simulink model "DFIG_FILTER"  (R2023a)
settings: Solver=ode23t  StartTime=0.0  StopTime=25  MaxStep=1e-6  RelTol=1e-3
model workspace (MAT data in the model file):
  Ts_phasor = 10
undefined symbols (not defined in the file): Base_Power, D1, Delta, F, find_system, Fnom, gcbh, H, ILd_init, ILq_init, Imax_grid_conv, Init, j, Ki_dc_reg, Ki_grid_side_cur_reg, Ki_power_reg, Ki_Q, Ki_rotor_side_cur_reg, Ki_volt_reg, Kp_dc_reg, Kp_grid_side_cur_reg, Kp_power_reg, Kp_Q, Kp_rotor_side_cur_reg, Kp_volt_reg, L_RL, Llr, Lls, p, Pnom, power_A, power_B, power_D, R_RL, Rr, Rs, speed_A, speed_B, speed_C, speed_D, sps_rtmsupport, Vcontrol, Vnom, Wind_On
libraries: spsPower3phPhasorLib x9, spsOnDelayLib x9, spsThreePhaseVIMeasurementLib x8, simulink_extras x5, spsRMSLib x4, spsControlledCurrentSourceLib x4, spsGroundLib x3, spsSeriesRLCBranchLib x2, spsThreePhaseSeriesRLCBranchLib x2, spspowerguiLib x2, spsThreePhasePISectionLineLib x2, spsThreePhaseTransformerTwoWindingsLib x2
(part 3 of 6)

== system DFIG_FILTER/MODEL (PHASER)/Wind turbine Data acquisition4/Mean Value2 ==
  note: Mean value
  In : Inport
  Init : Inport  Port=2
  Gain : Gain  Gain=1/Period  SaturateOnIntegerOverflow=on  OutDataTypeStr=Inherit: Same as input  ParamDataTypeStr=Inherit: Same as input
  Step : Step  Time=Period+eps  SampleTime=0
  Sum : Sum  Inputs=+-  InputSameDT=on  SaturateOnIntegerOverflow=on  OutDataTypeStr=Inherit: Same as first input
  Switch : Switch  Threshold=0.5  InputSameDT=off
  Transport Delay : TransportDelay  DelayTime=Period
  integrator : Integrator
  Mean : Outport  VectorParamsAs1DForOutWhenUnconnected=off
  wires:
  Init/1 -> Switch/3
  Step/1 -> Switch/2
  Switch/1 -> Mean/1
  Gain/1 -> Switch/1
  Sum/1 -> Gain/1
  In/1 -> integrator/1
  integrator/1 -> Sum/1, Transport Delay/1
  Transport Delay/1 -> Sum/2

== system DFIG_FILTER/MODEL (PHASER)/Wind turbine Data acquisition4/magnitude positive seq.  ==
  In1 : Inport
  Complex to Real-Imag : ComplexToRealImag
  Fourier1 : Subsystem  mask(Fourier analyser){f1=60, n=0}
      mask prompts: f1 "Fundamental frequency f1 (Hz):"; n "Harmonic n (0=DC; 1=fundamental; 2=2nd harm;  ...) :"
      mask help: The Fourier block performs a Fourier analysis of the input signal over a running window of one cycle of the fundamental frequency. First and second outputs return respectively the magnitude and phase (degrees) of the harmonic component specified.
      mask init:
      | k=2-(n==0);
      mask Help: helpview(psbhelp)
  Fourier2 : Subsystem  mask(Fourier analyser){f1=60, n=0}
      mask prompts: f1 "Fundamental frequency f1 (Hz):"; n "Harmonic n (0=DC; 1=fundamental; 2=2nd harm;  ...) :"
      mask help: The Fourier block performs a Fourier analysis of the input signal over a running window of one cycle of the fundamental frequency. First and second outputs return respectively the magnitude and phase (degrees) of the harmonic component specified.
      mask init:
      | k=2-(n==0);
      mask Help: helpview(psbhelp)
  Math Function : Math  Operator=hypot  SignedPower=on
  Terminator : Terminator
  Terminator1 : Terminator
  Out1 : Outport  VectorParamsAs1DForOutWhenUnconnected=off
  wires:
  In1/1 -> Complex to Real-Imag/1
  Math Function/1 -> Out1/1
  Fourier2/1(magnitude) -> Math Function/2
  Fourier1/1(magnitude) -> Math Function/1
  Fourier2/2(angle) -> Terminator1/1
  Fourier1/2(angle) -> Terminator/1
  Complex to Real-Imag/2 -> Fourier2/1(signal)
  Complex to Real-Imag/1 -> Fourier1/1(signal)

== system DFIG_FILTER/MODEL (PHASER)/Wind turbine Data acquisition4/magnitude positivie seq ==
  In1 : Inport
  Complex to Real-Imag : ComplexToRealImag
  Fourier1 : Subsystem  mask(Fourier analyser){f1=60, n=0}
      mask prompts: f1 "Fundamental frequency f1 (Hz):"; n "Harmonic n (0=DC; 1=fundamental; 2=2nd harm;  ...) :"
      mask help: The Fourier block performs a Fourier analysis of the input signal over a running window of one cycle of the fundamental frequency. First and second outputs return respectively the magnitude and phase (degrees) of the harmonic component specified.
      mask init:
      | k=2-(n==0);
      mask Help: helpview(psbhelp)
  Fourier2 : Subsystem  mask(Fourier analyser){f1=60, n=0}
      mask prompts: f1 "Fundamental frequency f1 (Hz):"; n "Harmonic n (0=DC; 1=fundamental; 2=2nd harm;  ...) :"
      mask help: The Fourier block performs a Fourier analysis of the input signal over a running window of one cycle of the fundamental frequency. First and second outputs return respectively the magnitude and phase (degrees) of the harmonic component specified.
      mask init:
      | k=2-(n==0);
      mask Help: helpview(psbhelp)
  Math Function : Math  Operator=hypot  SignedPower=on
  Terminator : Terminator
  Terminator1 : Terminator
  Out1 : Outport  VectorParamsAs1DForOutWhenUnconnected=off
  wires:
  Complex to Real-Imag/1 -> Fourier1/1(signal)
  Complex to Real-Imag/2 -> Fourier2/1(signal)
  Fourier1/2(angle) -> Terminator/1
  Fourier2/2(angle) -> Terminator1/1
  Fourier1/1(magnitude) -> Math Function/1
  Fourier2/1(magnitude) -> Math Function/2
  Math Function/1 -> Out1/1
  In1/1 -> Complex to Real-Imag/1

== system DFIG_FILTER/MODEL (PHASER)/Wind turbine Data acquisition5/Mean Value1 ==
  note: Mean value
  In : Inport
  Init : Inport  Port=2
  Gain : Gain  Gain=1/Period  SaturateOnIntegerOverflow=on  OutDataTypeStr=Inherit: Same as input  ParamDataTypeStr=Inherit: Same as input
  Step : Step  Time=Period+eps  SampleTime=0
  Sum : Sum  Inputs=+-  InputSameDT=on  SaturateOnIntegerOverflow=on  OutDataTypeStr=Inherit: Same as first input
  Switch : Switch  Threshold=0.5  InputSameDT=off
  Transport Delay : TransportDelay  DelayTime=Period
  integrator : Integrator
  Mean : Outport  VectorParamsAs1DForOutWhenUnconnected=off
  wires:
  Transport Delay/1 -> Sum/2
  integrator/1 -> Transport Delay/1, Sum/1
  In/1 -> integrator/1
  Sum/1 -> Gain/1
  Gain/1 -> Switch/1
  Switch/1 -> Mean/1
  Step/1 -> Switch/2
  Init/1 -> Switch/3

== system DFIG_FILTER/MODEL (PHASER)/Wind turbine Data acquisition5/Mean Value2 ==
  note: Mean value
  In : Inport
  Init : Inport  Port=2
  Gain : Gain  Gain=1/Period  SaturateOnIntegerOverflow=on  OutDataTypeStr=Inherit: Same as input  ParamDataTypeStr=Inherit: Same as input
  Step : Step  Time=Period+eps  SampleTime=0
  Sum : Sum  Inputs=+-  InputSameDT=on  SaturateOnIntegerOverflow=on  OutDataTypeStr=Inherit: Same as first input
  Switch : Switch  Threshold=0.5  InputSameDT=off
  Transport Delay : TransportDelay  DelayTime=Period
  integrator : Integrator
  Mean : Outport  VectorParamsAs1DForOutWhenUnconnected=off
  wires:
  Init/1 -> Switch/3
  Step/1 -> Switch/2
  Switch/1 -> Mean/1
  Gain/1 -> Switch/1
  Sum/1 -> Gain/1
  In/1 -> integrator/1
  integrator/1 -> Sum/1, Transport Delay/1
  Transport Delay/1 -> Sum/2

== system DFIG_FILTER/MODEL (PHASER)/Wind turbine Data acquisition5/magnitude positive seq.  ==
  In1 : Inport
  Complex to Real-Imag : ComplexToRealImag
  Fourier1 : Subsystem  mask(Fourier analyser){f1=60, n=0}
      mask prompts: f1 "Fundamental frequency f1 (Hz):"; n "Harmonic n (0=DC; 1=fundamental; 2=2nd harm;  ...) :"
      mask help: The Fourier block performs a Fourier analysis of the input signal over a running window of one cycle of the fundamental frequency. First and second outputs return respectively the magnitude and phase (degrees) of the harmonic component specified.
      mask init:
      | k=2-(n==0);
      mask Help: helpview(psbhelp)
  Fourier2 : Subsystem  mask(Fourier analyser){f1=60, n=0}
      mask prompts: f1 "Fundamental frequency f1 (Hz):"; n "Harmonic n (0=DC; 1=fundamental; 2=2nd harm;  ...) :"
      mask help: The Fourier block performs a Fourier analysis of the input signal over a running window of one cycle of the fundamental frequency. First and second outputs return respectively the magnitude and phase (degrees) of the harmonic component specified.
      mask init:
      | k=2-(n==0);
      mask Help: helpview(psbhelp)
  Math Function : Math  Operator=hypot  SignedPower=on
  Terminator : Terminator
  Terminator1 : Terminator
  Out1 : Outport  VectorParamsAs1DForOutWhenUnconnected=off
  wires:
  In1/1 -> Complex to Real-Imag/1
  Math Function/1 -> Out1/1
  Fourier2/1(magnitude) -> Math Function/2
  Fourier1/1(magnitude) -> Math Function/1
  Fourier2/2(angle) -> Terminator1/1
  Fourier1/2(angle) -> Terminator/1
  Complex to Real-Imag/2 -> Fourier2/1(signal)
  Complex to Real-Imag/1 -> Fourier1/1(signal)

== system DFIG_FILTER/MODEL (PHASER)/Wind turbine Data acquisition5/magnitude positivie seq ==
  In1 : Inport
  Complex to Real-Imag : ComplexToRealImag
  Fourier1 : Subsystem  mask(Fourier analyser){f1=60, n=0}
      mask prompts: f1 "Fundamental frequency f1 (Hz):"; n "Harmonic n (0=DC; 1=fundamental; 2=2nd harm;  ...) :"
      mask help: The Fourier block performs a Fourier analysis of the input signal over a running window of one cycle of the fundamental frequency. First and second outputs return respectively the magnitude and phase (degrees) of the harmonic component specified.
      mask init:
      | k=2-(n==0);
      mask Help: helpview(psbhelp)
  Fourier2 : Subsystem  mask(Fourier analyser){f1=60, n=0}
      mask prompts: f1 "Fundamental frequency f1 (Hz):"; n "Harmonic n (0=DC; 1=fundamental; 2=2nd harm;  ...) :"
      mask help: The Fourier block performs a Fourier analysis of the input signal over a running window of one cycle of the fundamental frequency. First and second outputs return respectively the magnitude and phase (degrees) of the harmonic component specified.
      mask init:
      | k=2-(n==0);
      mask Help: helpview(psbhelp)
  Math Function : Math  Operator=hypot  SignedPower=on
  Terminator : Terminator
  Terminator1 : Terminator
  Out1 : Outport  VectorParamsAs1DForOutWhenUnconnected=off
  wires:
  Complex to Real-Imag/1 -> Fourier1/1(signal)
  Complex to Real-Imag/2 -> Fourier2/1(signal)
  Fourier1/2(angle) -> Terminator/1
  Fourier2/2(angle) -> Terminator1/1
  Fourier1/1(magnitude) -> Math Function/1
  Fourier2/1(magnitude) -> Math Function/2
  Math Function/1 -> Out1/1
  In1/1 -> Complex to Real-Imag/1

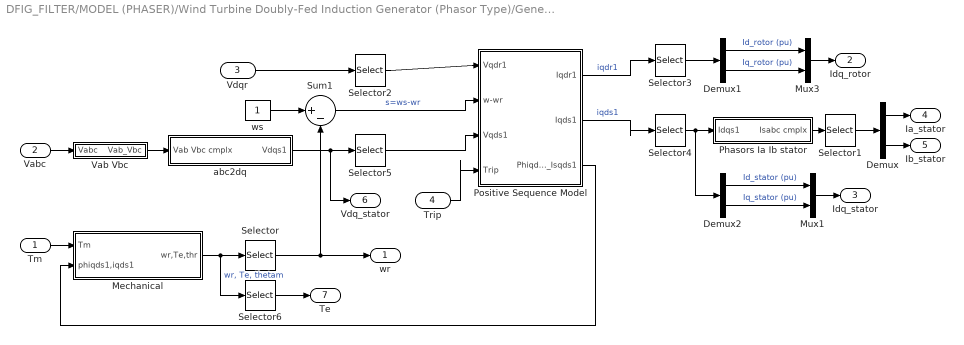
== system DFIG_FILTER/MODEL (PHASER)/Wind Turbine Doubly-Fed Induction Generator (Phasor Type)/Generator & Converters/Asynchronous machine Positive sequence phasor model Inputs and outputs are in per unit (pu) ==
  Tm : Inport
  Vabc : Inport  Port=2
  "Vdqr " : Inport  Port=3
  Trip : Inport  Port=4
  Demux : Demux  Outputs=2
      settings: DisplayOption=none
  Demux1 : Demux  Outputs=2
      settings: DisplayOption=none
  Demux2 : Demux  Outputs=2
      settings: DisplayOption=none
  Mechanical : Subsystem
  Mux1 : Mux  Inputs=2
  Mux3 : Mux  Inputs=2
  Phasors Ia Ib stator : Subsystem
  Positive Sequence Model : Subsystem
  Selector : Selector  InputPortWidth=3  IndexOptions=Index vector (dialog)  Indices=1  OutputSizes=1
  Selector1 : Selector  InputPortWidth=3  IndexOptions=Index vector (dialog)  Indices=[1 2]  OutputSizes=1
  Selector{2..5} (4 alike) : Selector  InputPortWidth=2  IndexOptions=Index vector (dialog)  Indices=[2 1]  OutputSizes=1
  Selector6 : Selector  InputPortWidth=3  IndexOptions=Index vector (dialog)  Indices=2  OutputSizes=1
  Sum1 : Sum  Inputs=|+-  InputSameDT=on  SaturateOnIntegerOverflow=on  OutDataTypeStr=Inherit: Same as first input
  Vab Vbc : Subsystem
  abc2dq : Subsystem
  ws : Constant
  wr : Outport  VectorParamsAs1DForOutWhenUnconnected=off
  Idq_rotor : Outport  Port=2  VectorParamsAs1DForOutWhenUnconnected=off
  Idq_stator : Outport  Port=3  VectorParamsAs1DForOutWhenUnconnected=off
  Ia_stator : Outport  Port=4  VectorParamsAs1DForOutWhenUnconnected=off
  Ib_stator : Outport  Port=5  VectorParamsAs1DForOutWhenUnconnected=off
  Vdq_stator : Outport  Port=6  VectorParamsAs1DForOutWhenUnconnected=off
  Te : Outport  Port=7  VectorParamsAs1DForOutWhenUnconnected=off
  wires:
  Selector4/1 -> Phasors Ia Ib stator/1(Idqs1), Demux2/1
  Selector5/1 -> Positive Sequence Model/3(Vqds1)
  Selector2/1 -> Positive Sequence Model/1(Vqdr1)
  Sum1/1 -> Positive Sequence Model/2(w-wr)  "s=ws-wr"
  Selector/1 -> wr/1, Sum1/2
  ws/1 -> Sum1/1
  Mechanical/1(wr,Te,thr) -> Selector/1, Selector6/1  "wr, Te, thetam"
  "Vdqr "/1 -> Selector2/1
  abc2dq/1(Vdqs1) -> Selector5/1, Vdq_stator/1
  Vab Vbc/1(Vab_Vbc) -> abc2dq/1(Vab Vbc cmplx)
  Vabc/1 -> Vab Vbc/1(Vabc)
  Phasors Ia Ib stator/1(Isabc cmplx) -> Selector1/1
  Tm/1 -> Mechanical/1(Tm)
  Demux/1 -> Ia_stator/1
  Demux/2 -> Ib_stator/1
  Selector1/1 -> Demux/1
  Selector6/1 -> Te/1
  Selector3/1 -> Demux1/1
  Demux1/1 -> Mux3/1  "Id_rotor (pu)"
  Demux1/2 -> Mux3/2  "Iq_rotor (pu)"
  Mux3/1 -> Idq_rotor/1
  Demux2/1 -> Mux1/1  "Id_stator (pu)"
  Demux2/2 -> Mux1/2  "Iq_stator (pu)"
  Mux1/1 -> Idq_stator/1
  Positive Sequence Model/1(Iqdr1) -> Selector3/1  "iqdr1"
  Positive Sequence Model/2(Iqds1) -> Selector4/1  "iqds1"
  Positive Sequence Model/3(Phiqds1_Isqds1) -> Mechanical/2(phiqds1,iqds1)
  Trip/1 -> Positive Sequence Model/4(Trip)

== system DFIG_FILTER/MODEL (PHASER)/Wind Turbine Doubly-Fed Induction Generator (Phasor Type)/Generator & Converters/Control ==
  Vabc_B1 : Inport
  Idq_grid_conv : Inport  Port=2
  Vdc : Inport  Port=3
  wr : Inport  Port=4
  Idq_stator : Inport  Port=5
  Idq_rotor : Inport  Port=6
  V_ref : Inport  Port=7  SampleTime=0
  Q_ref : Inport  Port=8  SampleTime=0
  Iq_grid_conv_ref : Inport  Port=9  SampleTime=0
  P_B1 : Inport  Port=10
  Q_B1 : Inport  Port=11
  Trip : Inport  Port=12
  0-inf : Saturate  UpperLimit=inf  LowerLimit=0
  0-pitch_max : Saturate  UpperLimit=pitch_max  LowerLimit=0
  Constant2 : Constant  Value=speed_D
  Converters voltages : Subsystem
  Logical Operator : Logic  Operator=NOT  AllPortsSameDT=off  OutDataTypeStr=float('double')  SampleTime=0
  Power(speed) : Lookup_n-D  NumberOfTableDimensions=1  BreakpointsForDimension1=speed_power(:,1)  Table=speed_power(:,2)  InternalRulePriority=Speed  RndMeth=Simplest
  "Rate Limiter " : RateLimiter  RisingSlewLimit=power_slew_rate  FallingSlewLimit=-power_slew_rate
  "Rate Limiter   " : RateLimiter  RisingSlewLimit=pitch_rate  FallingSlewLimit=-pitch_rate
  Sum : Sum  Inputs=|+-  SaturateOnIntegerOverflow=on
  abc2dq & Positive sequence Voltage phase angle : Subsystem
  pitch_gain : Gain  Gain=pitch_gain  SaturateOnIntegerOverflow=on  OutDataTypeStr=Inherit: Same as input  ParamDataTypeStr=Inherit: Same as input
  wind_dfig_grid : Subsystem
  wind_dfig_rotor : Subsystem
  Vdq_rotor_conv : Outport  VectorParamsAs1DForOutWhenUnconnected=off
  Vdq_B1 : Outport  Port=2  VectorParamsAs1DForOutWhenUnconnected=off
  Vdq_grid_conv : Outport  Port=3  VectorParamsAs1DForOutWhenUnconnected=off
  Pitch_angle : Outport  Port=4  VectorParamsAs1DForOutWhenUnconnected=off
  wires:
  Vdc/1 -> Converters voltages/2(Vdc), wind_dfig_grid/4(Vdc), wind_dfig_rotor/2(Vdc)
  abc2dq & Positive sequence Voltage phase angle/2(Theta) -> wind_dfig_grid/3(Theta), wind_dfig_rotor/3(Theta)
  abc2dq & Positive sequence Voltage phase angle/1(Vdq_B1) -> Vdq_B1/1, wind_dfig_grid/1(Vdq_B1)
  Converters voltages/2(Vdq_rotor_conv) -> Vdq_rotor_conv/1
  Converters voltages/1(Vdq_grid_conv) -> Vdq_grid_conv/1
  Idq_grid_conv/1 -> wind_dfig_grid/2(Idq_grid_conv), wind_dfig_rotor/11(Idq_grid_conv)
  Vabc_B1/1 -> abc2dq & Positive sequence Voltage phase angle/1(Vabc_B1)
  Iq_grid_conv_ref/1 -> wind_dfig_grid/5(Iq_ref)
  Idq_stator/1 -> wind_dfig_rotor/4(Idq_stator)
  Idq_rotor/1 -> wind_dfig_rotor/5(Idq_rotor)
  V_ref/1 -> wind_dfig_rotor/6(V_ref)
  Q_ref/1 -> wind_dfig_rotor/7(Q_ref)
  abc2dq & Positive sequence Voltage phase angle/3(V_B1) -> wind_dfig_rotor/8(V_B1)
  wr/1 -> Power(speed)/1, Sum/1, wind_dfig_rotor/1(wr)
  P_B1/1 -> wind_dfig_rotor/9(P_B1)
  Q_B1/1 -> wind_dfig_rotor/10(Q_B1)
  Trip/1 -> Logical Operator/1
  wind_dfig_grid/1(Vdq_ctrl_grid_conv) -> Converters voltages/1(Vdq_ctrl_grid_conv)
  0-inf/1 -> "Rate Limiter "/1
  Power(speed)/1 -> 0-inf/1
  "Rate Limiter "/1 -> wind_dfig_rotor/12(Power_opt)
  0-pitch_max/1 -> "Rate Limiter   "/1
  Constant2/1 -> Sum/2
  Sum/1 -> pitch_gain/1
  pitch_gain/1 -> 0-pitch_max/1
  "Rate Limiter   "/1 -> Pitch_angle/1
  wind_dfig_rotor/1(Vdq_ctrl_rotor_conv) -> Converters voltages/3(Vdq_ctrl_rotor_conv)
  Logical Operator/1 -> wind_dfig_grid/Enable, wind_dfig_rotor/Enable

== system DFIG_FILTER/MODEL (PHASER)/Wind Turbine Doubly-Fed Induction Generator (Phasor Type)/Generator & Converters/DC bus model ==
  note: Pdc = Pac_grid_conv - Pac_rotor_conv
  Pac_grid_conv : Inport
  Pac_rotor_conv : Inport  Port=2
  Integrator : Integrator  InitialCondition=Vdc_Init  LowerSaturationLimit=1e-6  ZeroCross=off
  Product2 : Product  Inputs=*/  InputSameDT=on  SaturateOnIntegerOverflow=on  OutDataTypeStr=Inherit: Same as first input
  Sum2 : Sum  Inputs=|+-  InputSameDT=on  SaturateOnIntegerOverflow=on  OutDataTypeStr=Inherit: Same as first input
  deg->rad1 : Gain  Gain=1/C  SaturateOnIntegerOverflow=on  OutDataTypeStr=Inherit: Same as input  ParamDataTypeStr=Inherit: Same as input
  pu->W : Gain  Gain=Pnom  SaturateOnIntegerOverflow=on  OutDataTypeStr=Inherit: Same as input  ParamDataTypeStr=Inherit: Same as input
  Vdc : Outport  VectorParamsAs1DForOutWhenUnconnected=off
  wires:
  pu->W/1 -> Product2/1
  Pac_grid_conv/1 -> Sum2/1
  deg->rad1/1 -> Integrator/1
  Integrator/1 -> Vdc/1, Product2/2  "Vdc"
  Product2/1 -> deg->rad1/1  "Idc"
  Pac_rotor_conv/1 -> Sum2/2
  Sum2/1 -> pu->W/1

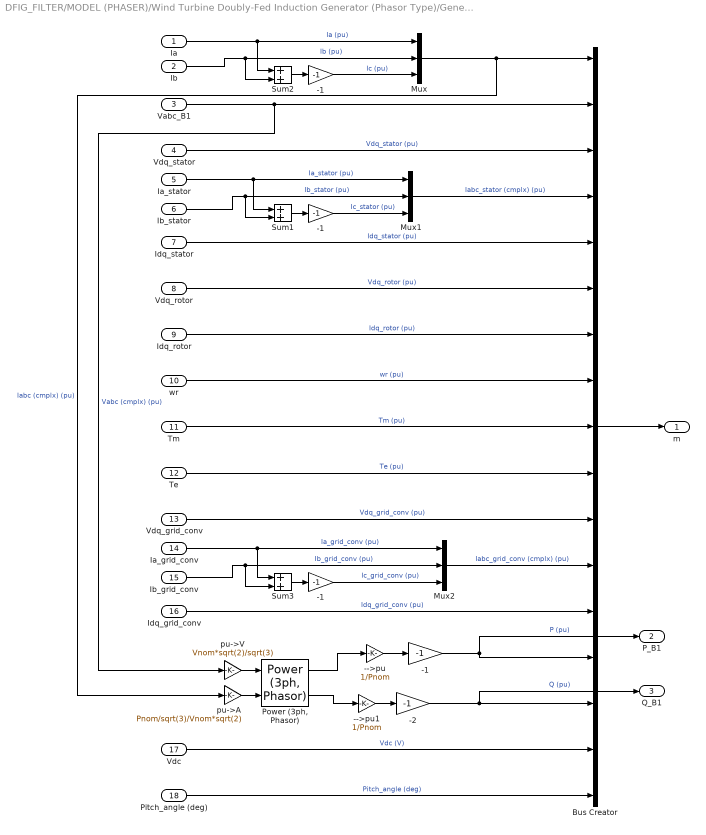
== system DFIG_FILTER/MODEL (PHASER)/Wind Turbine Doubly-Fed Induction Generator (Phasor Type)/Generator & Converters/Data acquisition ==
  Ia : Inport
  Ib : Inport  Port=2
  Vabc_B1 : Inport  Port=3
  Vdq_stator : Inport  Port=4
  Ia_stator : Inport  Port=5
  Ib_stator : Inport  Port=6
  Idq_stator : Inport  Port=7
  Vdq_rotor : Inport  Port=8
  Idq_rotor : Inport  Port=9
  wr : Inport  Port=10
  Tm : Inport  Port=11
  Te : Inport  Port=12
  Vdq_grid_conv : Inport  Port=13
  Ia_grid_conv : Inport  Port=14
  Ib_grid_conv : Inport  Port=15
  Idq_grid_conv : Inport  Port=16
  Vdc : Inport  Port=17
  Pitch_angle (deg) : Inport  Port=18
  " -1" : Gain  Gain=-1  SaturateOnIntegerOverflow=on  OutDataTypeStr=Inherit: Same as input  ParamDataTypeStr=Inherit: Same as input
  -->pu : Gain  Gain=1/Pnom  SaturateOnIntegerOverflow=on  OutDataTypeStr=Inherit: Same as input  ParamDataTypeStr=Inherit: Same as input
  -->pu1 : Gain  Gain=1/Pnom  SaturateOnIntegerOverflow=on  OutDataTypeStr=Inherit: Same as input  ParamDataTypeStr=Inherit: Same as input
  -1 : Gain  Gain=-1  SaturateOnIntegerOverflow=on  OutDataTypeStr=Inherit: Same as input  ParamDataTypeStr=Inherit: Same as input
  "-1 " : Gain  Gain=-1  SaturateOnIntegerOverflow=on  OutDataTypeStr=Inherit: Same as input  ParamDataTypeStr=Inherit: Same as input
  "-1  " : Gain  Gain=-1  SaturateOnIntegerOverflow=on  OutDataTypeStr=Inherit: Same as input  ParamDataTypeStr=Inherit: Same as input
  -2 : Gain  Gain=-1  SaturateOnIntegerOverflow=on  OutDataTypeStr=Inherit: Same as input  ParamDataTypeStr=Inherit: Same as input
  Bus Creator : BusCreator  Inputs=17
  Mux : Mux  Inputs=3
  Mux1 : Mux  Inputs=3
  Mux2 : Mux  Inputs=3
  "Power (3ph, Phasor)" : spsPower3phPhasorLib/Power (3ph, Phasor)
      settings: LibrarySourceBlock=|
      | sps_lib/Sensors and Measurements/Power
      | (3ph, Phasor)
  Sum1 : Sum  SaturateOnIntegerOverflow=on
  Sum2 : Sum  SaturateOnIntegerOverflow=on
  Sum3 : Sum  SaturateOnIntegerOverflow=on
  pu->A : Gain  Gain=Pnom/sqrt(3)/Vnom*sqrt(2)  SaturateOnIntegerOverflow=on  OutDataTypeStr=Inherit: Same as input  ParamDataTypeStr=Inherit: Same as input
  pu->V : Gain  Gain=Vnom*sqrt(2)/sqrt(3)  SaturateOnIntegerOverflow=on  OutDataTypeStr=Inherit: Same as input  ParamDataTypeStr=Inherit: Same as input
  m : Outport  VectorParamsAs1DForOutWhenUnconnected=off
  P_B1 : Outport  Port=2  VectorParamsAs1DForOutWhenUnconnected=off
  Q_B1 : Outport  Port=3  VectorParamsAs1DForOutWhenUnconnected=off
  wires:
  pu->A/1 -> "Power (3ph, Phasor)"/2
  -->pu/1 -> -1/1
  Sum2/1 -> "-1 "/1
  "-1 "/1 -> Mux/3  "Ic (pu)"
  Ib/1 -> Sum2/2, Mux/2  "Ib (pu)"
  Ia/1 -> Sum2/1, Mux/1  "Ia (pu)"
  Sum1/1 -> "-1  "/1
  "-1  "/1 -> Mux1/3  "Ic_stator (pu)"
  Ib_stator/1 -> Mux1/2, Sum1/2  "Ib_stator (pu)"
  Ia_stator/1 -> Mux1/1, Sum1/1  "Ia_stator (pu)"
  pu->V/1 -> "Power (3ph, Phasor)"/1
  Sum3/1 -> " -1"/1
  " -1"/1 -> Mux2/3  "Ic_grid_conv (pu)"
  Ib_grid_conv/1 -> Sum3/2, Mux2/2  "Ib_grid_conv (pu)"
  Ia_grid_conv/1 -> Sum3/1, Mux2/1  "Ia_grid_conv (pu)"
  Mux1/1 -> Bus Creator/4  "Iabc_stator (cmplx) (pu)"
  Mux/1 -> pu->A/1, Bus Creator/1  "Iabc (cmplx) (pu)"
  Vabc_B1/1 -> pu->V/1, Bus Creator/2  "Vabc (cmplx) (pu)"
  Vdq_stator/1 -> Bus Creator/3  "Vdq_stator (pu)"
  Idq_stator/1 -> Bus Creator/5  "Idq_stator (pu)"
  Vdq_rotor/1 -> Bus Creator/6  "Vdq_rotor (pu)"
  Idq_rotor/1 -> Bus Creator/7  "Idq_rotor (pu)"
  wr/1 -> Bus Creator/8  "wr (pu)"
  Tm/1 -> Bus Creator/9  "Tm (pu)"
  Te/1 -> Bus Creator/10  "Te (pu)"
  Vdq_grid_conv/1 -> Bus Creator/11  "Vdq_grid_conv (pu)"
  Mux2/1 -> Bus Creator/12  "Iabc_grid_conv (cmplx) (pu)"
  Idq_grid_conv/1 -> Bus Creator/13  "Idq_grid_conv (pu)"
  Vdc/1 -> Bus Creator/16  "Vdc (V)"
  -2/1 -> Q_B1/1, Bus Creator/15  "Q (pu)"
  -1/1 -> Bus Creator/14, P_B1/1  "P (pu)"
  Pitch_angle (deg)/1 -> Bus Creator/17  "Pitch_angle (deg)"
  Bus Creator/1 -> m/1
  -->pu1/1 -> -2/1
  "Power (3ph, Phasor)"/1 -> -->pu/1
  "Power (3ph, Phasor)"/2 -> -->pu1/1

== system DFIG_FILTER/MODEL (PHASER)/Wind Turbine Doubly-Fed Induction Generator (Phasor Type)/Generator & Converters/Grid-side converter currents & Converters power ==
  Vdq_rotor_conv : Inport
  Vdq_B1 : Inport  Port=2
  Vdq_grid_conv : Inport  Port=3
  Idq_rotor_conv : Inport  Port=4
  Trip : Inport  Port=5
  Demux : Demux  Outputs=2
      settings: DisplayOption=none
  Demux1 : Demux  Outputs=2
      settings: DisplayOption=none
  Mux2 : Mux  Inputs=2
  Product1 : Product  Inputs=**  InputSameDT=on  SaturateOnIntegerOverflow=on  OutDataTypeStr=Inherit: Same as first input
  Product3 : Product  Inputs=**  InputSameDT=on  SaturateOnIntegerOverflow=on  OutDataTypeStr=Inherit: Same as first input
  Sum1 : Sum  Inputs=1  InputSameDT=on  SaturateOnIntegerOverflow=on  OutDataTypeStr=Inherit: Same as first input
  Sum3 : Sum  Inputs=1  InputSameDT=on  SaturateOnIntegerOverflow=on  OutDataTypeStr=Inherit: Same as first input
  d-q axis model of a 3-phase series R-L branch : Subsystem  mask(d-q axis model of a 3-phase series R-L branch){R=R_RL, L=L_RL, Fnom=Fnom, Idq0=[ILd_init ILq_init]}
      mask prompts: R "R (pu)"; L "L (pu)"; Fnom "Nominal frequency (Hz)"; Idq0 "Initial currents [Id Iq] (pu)"
      mask help:
      | This block implements a d-q axis model of a 3-phase R-L branch.
      | Inputs:
      | d-q axis voltages (V1 and V2) at each terminal of the R-L branch in pu.
      | Outputs:
      | d-q axis currents flowing (from V1 to V2) in the R-L branch in pu.
      mask init:
      | w=2*pi*Fnom;
  dq2ab : Subsystem
  Ia_grid_conv : Outport  VectorParamsAs1DForOutWhenUnconnected=off
  Ib_grid_conv : Outport  Port=2  VectorParamsAs1DForOutWhenUnconnected=off
  Idq_grid_conv : Outport  Port=3  VectorParamsAs1DForOutWhenUnconnected=off
  Pac_grid_conv : Outport  Port=4  VectorParamsAs1DForOutWhenUnconnected=off
  Pac_rotor_conv : Outport  Port=5  VectorParamsAs1DForOutWhenUnconnected=off
  wires:
  Demux/2 -> Ib_grid_conv/1
  Demux/1 -> Ia_grid_conv/1
  dq2ab/1(Ia_Ib complx) -> Demux/1
  d-q axis model of a 3-phase series R-L branch/1(Idq) -> dq2ab/1(Idq_seq1), Demux1/1, Product3/1
  Idq_rotor_conv/1 -> Product1/2
  Vdq_rotor_conv/1 -> Product1/1
  Sum1/1 -> Pac_rotor_conv/1
  Product1/1 -> Sum1/1
  Sum3/1 -> Pac_grid_conv/1
  Product3/1 -> Sum3/1
  Vdq_grid_conv/1 -> d-q axis model of a 3-phase series R-L branch/2(Vdq2), Product3/2
  Vdq_B1/1 -> d-q axis model of a 3-phase series R-L branch/1(Vdq1)
  Demux1/1 -> Mux2/1  "Id_grid_conv (pu)"
  Demux1/2 -> Mux2/2  "Iq_grid_conv (pu)"
  Mux2/1 -> Idq_grid_conv/1
  Trip/1 -> d-q axis model of a 3-phase series R-L branch/3(Trip)

== system DFIG_FILTER/MODEL (PHASER)/Wind Turbine Protection/Protection System/AC Current Protection ==
  abc : Inport  PortDimensions=3
  Complex to Magnitude-Angle1 : ComplexToMagnitudeAngle  Output=Magnitude
  Current Measurement : Subsystem
  MinMax : MinMax  Function=max  InputSameDT=on  SaturateOnIntegerOverflow=on  ZeroCross=off
  Mux : Mux  Inputs=3
  On Delay : spsOnDelayLib/On Delay  DelayType=On delay  delay=Delay_I1  ic=0  Ts=0
  On Delay1 : spsOnDelayLib/On Delay  DelayType=On delay  delay=Delay_I2_I1  ic=0  Ts=0
  Relational Operator10 : RelationalOperator  Operator=>  InputSameDT=off
  Relational Operator6 : RelationalOperator  Operator=>  InputSameDT=off
  Relational Operator8 : RelationalOperator  Operator=>  InputSameDT=off
  Selector : Selector  InputPortWidth=3  IndexOptions=Index vector (dialog)  Indices=1  OutputSizes=1
  Selector1 : Selector  InputPortWidth=3  IndexOptions=Index vector (dialog)  Indices=2  OutputSizes=1
  Selector2 : Selector  InputPortWidth=3  IndexOptions=Index vector (dialog)  Indices=3  OutputSizes=1
  V0/V1 max3 : Constant  Value=Max_I1
  V1 max : Constant  Value=Max_I2_I1
  V1 max2 : Constant  Value=Max_Iinst
  MaxIinst : Outport  VectorParamsAs1DForOutWhenUnconnected=off
  MaxI1 : Outport  Port=2  VectorParamsAs1DForOutWhenUnconnected=off
  MaxI2I1 : Outport  Port=3  VectorParamsAs1DForOutWhenUnconnected=off
  wires:
  abc/1 -> Current Measurement/1(abc), Selector/1, Selector1/1, Selector2/1
  Current Measurement/1(I1) -> Relational Operator6/1
  V0/V1 max3/1 -> Relational Operator6/2
  V1 max/1 -> Relational Operator8/2
  Current Measurement/2(I2/I1) -> Relational Operator8/1
  Relational Operator6/1 -> On Delay/1
  Relational Operator8/1 -> On Delay1/1
  On Delay/1 -> MaxI1/1
  On Delay1/1 -> MaxI2I1/1
  Relational Operator10/1 -> MaxIinst/1
  V1 max2/1 -> Relational Operator10/2
  Selector/1 -> Mux/1
  Selector2/1 -> Mux/3
  Selector1/1 -> Mux/2
  Mux/1 -> Complex to Magnitude-Angle1/1
  Complex to Magnitude-Angle1/1 -> MinMax/1
  MinMax/1 -> Relational Operator10/1

== system DFIG_FILTER/MODEL (PHASER)/Wind Turbine Protection/Protection System/AC Voltage Protection ==
  abc : Inport  PortDimensions=3
  On Delay : spsOnDelayLib/On Delay  DelayType=On delay  delay=Delay_V1  ic=0  Ts=0
  On Delay1 : spsOnDelayLib/On Delay  DelayType=On delay  delay=Delay_V2_V1  ic=0  Ts=0
  On Delay2 : spsOnDelayLib/On Delay  DelayType=On delay  delay=Delay_V1  ic=0  Ts=0
  On Delay3 : spsOnDelayLib/On Delay  DelayType=On delay  delay=Delay_V2_V1  ic=0  Ts=0
  Relational Operator6 : RelationalOperator  Operator=>  InputSameDT=off
  Relational Operator7 : RelationalOperator  Operator=<  InputSameDT=off
  Relational Operator8 : RelationalOperator  Operator=>  InputSameDT=off
  Relational Operator9 : RelationalOperator  Operator=>  InputSameDT=off
  V0/V1 max3 : Constant  Value=Max_V1
  V0/V1 max4 : Constant  Value=Min_V1
  V1 max : Constant  Value=Max_V2_V1
  V1 max1 : Constant  Value=Max_V0_V1
  Voltage Measurement : Subsystem
  MinV1 : Outport  VectorParamsAs1DForOutWhenUnconnected=off
  MaxV1 : Outport  Port=2  VectorParamsAs1DForOutWhenUnconnected=off
  MaxV2V1 : Outport  Port=3  VectorParamsAs1DForOutWhenUnconnected=off
  MaxV0V1 : Outport  Port=4  VectorParamsAs1DForOutWhenUnconnected=off
  wires:
  On Delay3/1 -> MaxV0V1/1
  On Delay1/1 -> MaxV2V1/1
  On Delay/1 -> MinV1/1
  On Delay2/1 -> MaxV1/1
  Relational Operator9/1 -> On Delay3/1
  Relational Operator8/1 -> On Delay1/1
  Relational Operator7/1 -> On Delay/1
  Relational Operator6/1 -> On Delay2/1
  Voltage Measurement/3(V0/V1) -> Relational Operator9/1
  V1 max1/1 -> Relational Operator9/2
  Voltage Measurement/2(V2/V1) -> Relational Operator8/1
  V1 max/1 -> Relational Operator8/2
  V0/V1 max4/1 -> Relational Operator7/2
  V0/V1 max3/1 -> Relational Operator6/2
  Voltage Measurement/1(V1) -> Relational Operator7/1, Relational Operator6/1
  abc/1 -> Voltage Measurement/1(abc)

== system DFIG_FILTER/MODEL (PHASER)/Wind Turbine Protection/Protection System/DC Voltage Protection ==
  Vdc : Inport
  On Delay : spsOnDelayLib/On Delay  DelayType=On delay  delay=Delay_Vdc  ic=0  Ts=0
  Relational Operator1 : RelationalOperator  Operator=>  InputSameDT=off
  V1 max3 : Constant  Value=Max_Vdc
  MaxVdc : Outport  VectorParamsAs1DForOutWhenUnconnected=off
  wires:
  Vdc/1 -> Relational Operator1/1
  V1 max3/1 -> Relational Operator1/2
  Relational Operator1/1 -> On Delay/1
  On Delay/1 -> MaxVdc/1

== system DFIG_FILTER/MODEL (PHASER)/Wind Turbine Protection/Protection System/Decoding ==
  Code : Inport
  Constant : Constant  Value=pow2(0:-1:-9)
  Constant6 : Constant  Value=2
  Math Function : Math  Operator=rem  SignedPower=on
  Product : Product  InputSameDT=on  SaturateOnIntegerOverflow=on  OutDataTypeStr=Inherit: Same as first input
  Rounding Function : Rounding
  Out : Outport  VectorParamsAs1DForOutWhenUnconnected=off
  wires:
  Constant/1 -> Product/2
  Code/1 -> Product/1
  Product/1 -> Rounding Function/1
  Constant6/1 -> Math Function/2
  Rounding Function/1 -> Math Function/1
  Math Function/1 -> Out/1

== system DFIG_FILTER/MODEL (PHASER)/Wind Turbine Protection/Protection System/Encoding ==
  In1 : Inport
  In2 : Inport  Port=2
  In3 : Inport  Port=3
  In4 : Inport  Port=4
  In5 : Inport  Port=5
  In6 : Inport  Port=6
  In7 : Inport  Port=7
  In8 : Inport  Port=8
  In9 : Inport  Port=9
  In10 : Inport  Port=10
  Constant12 : Constant  Value=pow2(0:1:9)
  Data Type Conversion : DataTypeConversion
  Mux : Mux  Inputs=10
  Product : Product  InputSameDT=on  SaturateOnIntegerOverflow=on  OutDataTypeStr=Inherit: Same as first input
  Sum : Sum  Inputs=1  InputSameDT=on  SaturateOnIntegerOverflow=on  OutDataTypeStr=Inherit: Same as first input
  Code : Outport  VectorParamsAs1DForOutWhenUnconnected=off
  wires:
  Data Type Conversion/1 -> Product/1
  Mux/1 -> Data Type Conversion/1
  In2/1 -> Mux/2
  In3/1 -> Mux/3
  In4/1 -> Mux/4
  In5/1 -> Mux/5
  In6/1 -> Mux/6
  In7/1 -> Mux/7
  In8/1 -> Mux/8
  In9/1 -> Mux/9
  In10/1 -> Mux/10
  In1/1 -> Mux/1
  Product/1 -> Sum/1
  Constant12/1 -> Product/2
  Sum/1 -> Code/1

== system DFIG_FILTER/MODEL (PHASER)/Wind Turbine Protection/Protection System/Sample & Hold ==
  note: Silvano Casoria
      | Power System Simulation Laboratory
      | IREQ, Hydro-Quebc
  note: Sample and Hold
  In : Inport
  S : Inport  Port=2
  IC=ic : Memory  InitialCondition=ic  InheritSampleTime=on
  Switch : Switch  Threshold=0.5
  "   " : Outport  InitialOutput=0  VectorParamsAs1DForOutWhenUnconnected=off
  wires:
  S/1 -> Switch/2
  In/1 -> Switch/1
  IC=ic/1 -> Switch/3
  Switch/1 -> IC=ic/1, "   "/1

== system DFIG_FILTER/MODEL (PHASER)/Wind Turbine Protection/Protection System/Sample & Hold1 ==
  note: Silvano Casoria
      | Power System Simulation Laboratory
      | IREQ, Hydro-Quebc
  note: Sample and Hold
  In : Inport
  S : Inport  Port=2
  IC=ic : Memory  InitialCondition=ic  InheritSampleTime=on
  Switch : Switch  Threshold=0.5
  "   " : Outport  InitialOutput=0  VectorParamsAs1DForOutWhenUnconnected=off
  wires:
  S/1 -> Switch/2
  In/1 -> Switch/1
  IC=ic/1 -> Switch/3
  Switch/1 -> IC=ic/1, "   "/1

== system DFIG_FILTER/MODEL (PHASER)/Wind Turbine Protection/Protection System/Under//Over Speed Protection ==
  Speed : Inport  PortDimensions=1
  On Delay : spsOnDelayLib/On Delay  DelayType=On delay  delay=Delay_Speed  ic=0  Ts=0
  On Delay1 : spsOnDelayLib/On Delay  DelayType=On delay  delay=Delay_Speed  ic=0  Ts=0
  Relational Operator1 : RelationalOperator  Operator=>  InputSameDT=off
  Relational Operator3 : RelationalOperator  Operator=<  InputSameDT=off
  V1 max1 : Constant  Value=Min_Speed
  V1 max3 : Constant  Value=Max_Speed
  MinSpeed : Outport  VectorParamsAs1DForOutWhenUnconnected=off
  MaxSpeed : Outport  Port=2  VectorParamsAs1DForOutWhenUnconnected=off
  wires:
  Relational Operator3/1 -> On Delay/1
  Relational Operator1/1 -> On Delay1/1
  V1 max1/1 -> Relational Operator3/2
  V1 max3/1 -> Relational Operator1/2
  Speed/1 -> Relational Operator3/1, Relational Operator1/1
  On Delay/1 -> MinSpeed/1
  On Delay1/1 -> MaxSpeed/1

== system DFIG_FILTER/MODEL (PHASER)/Wind turbine Data acquisition/magnitude positive seq. /Fourier1 ==
  signal : Inport
  Constant : Constant  Value=0
  Fcn : Fcn  Expr=u^2
  Fcn1 : Fcn  Expr=u^2
  Fcn2 : Fcn  Expr=sqrt(u)
  Fcn3 : Fcn  Expr=180/pi*atan2(u[2],u[1])
  Gain1 : Gain  Gain=k*f1  SaturateOnIntegerOverflow=on  OutDataTypeStr=Inherit: Same as input  ParamDataTypeStr=Inherit: Same as input
  Integ2 : Integrator  InitialConditionSource=external
  Mux : Mux  Inputs=2
  Product : Product  InputSameDT=on  SaturateOnIntegerOverflow=on  OutDataTypeStr=Inherit: Same as first input
  Product1 : Product  InputSameDT=on  SaturateOnIntegerOverflow=on  OutDataTypeStr=Inherit: Same as first input
  Sum : Sum  InputSameDT=on  SaturateOnIntegerOverflow=on  OutDataTypeStr=Inherit: Same as first input
  Sum1 : Sum  Inputs=+-  InputSameDT=on  SaturateOnIntegerOverflow=on  OutDataTypeStr=Inherit: Same as first input
  Sum2 : Sum  Inputs=+-  InputSameDT=on  SaturateOnIntegerOverflow=on  OutDataTypeStr=Inherit: Same as first input
  T : TransportDelay  DelayTime=1/f1  BufferSize=2048
  T1 : TransportDelay  DelayTime=1/f1  BufferSize=2048
  cos(nwt) : Sin  Frequency=2*pi*n*f1  Phase=pi/2  SampleTime=0
  integ1 : Integrator  InitialConditionSource=external
  sin(nwt) : Sin  Frequency=2*pi*n*f1  SampleTime=0
  magnitude : Outport  InitialOutput=0  VectorParamsAs1DForOutWhenUnconnected=off
  angle : Outport  Port=2  InitialOutput=0  VectorParamsAs1DForOutWhenUnconnected=off
  wires:
  Constant/1 -> integ1/2, Integ2/2
  Sum/1 -> Fcn2/1
  Fcn/1 -> Sum/1
  Fcn1/1 -> Sum/2
  Mux/1 -> Fcn3/1
  Fcn3/1 -> angle/1
  sin(nwt)/1 -> Product/1
  cos(nwt)/1 -> Product1/2
  Product/1 -> integ1/1
  Product1/1 -> Integ2/1
  T/1 -> Sum1/2
  T1/1 -> Sum2/2
  integ1/1 -> Sum1/1, T/1
  Integ2/1 -> T1/1, Sum2/1
  Sum2/1 -> Fcn1/1, Mux/2
  Sum1/1 -> Fcn/1, Mux/1
  signal/1 -> Gain1/1
  Gain1/1 -> Product/2, Product1/1
  Fcn2/1 -> magnitude/1

== system DFIG_FILTER/MODEL (PHASER)/Wind turbine Data acquisition/magnitude positive seq. /Fourier2 ==
  signal : Inport
  Constant : Constant  Value=0
  Fcn : Fcn  Expr=u^2
  Fcn1 : Fcn  Expr=u^2
  Fcn2 : Fcn  Expr=sqrt(u)
  Fcn3 : Fcn  Expr=180/pi*atan2(u[2],u[1])
  Gain1 : Gain  Gain=k*f1  SaturateOnIntegerOverflow=on  OutDataTypeStr=Inherit: Same as input  ParamDataTypeStr=Inherit: Same as input
  Integ2 : Integrator  InitialConditionSource=external
  Mux : Mux  Inputs=2
  Product : Product  InputSameDT=on  SaturateOnIntegerOverflow=on  OutDataTypeStr=Inherit: Same as first input
  Product1 : Product  InputSameDT=on  SaturateOnIntegerOverflow=on  OutDataTypeStr=Inherit: Same as first input
  Sum : Sum  InputSameDT=on  SaturateOnIntegerOverflow=on  OutDataTypeStr=Inherit: Same as first input
  Sum1 : Sum  Inputs=+-  InputSameDT=on  SaturateOnIntegerOverflow=on  OutDataTypeStr=Inherit: Same as first input
  Sum2 : Sum  Inputs=+-  InputSameDT=on  SaturateOnIntegerOverflow=on  OutDataTypeStr=Inherit: Same as first input
  T : TransportDelay  DelayTime=1/f1  BufferSize=2048
  T1 : TransportDelay  DelayTime=1/f1  BufferSize=2048
  cos(nwt) : Sin  Frequency=2*pi*n*f1  Phase=pi/2  SampleTime=0
  integ1 : Integrator  InitialConditionSource=external
  sin(nwt) : Sin  Frequency=2*pi*n*f1  SampleTime=0
  magnitude : Outport  InitialOutput=0  VectorParamsAs1DForOutWhenUnconnected=off
  angle : Outport  Port=2  InitialOutput=0  VectorParamsAs1DForOutWhenUnconnected=off
  wires:
  Fcn2/1 -> magnitude/1
  Gain1/1 -> Product1/1, Product/2
  signal/1 -> Gain1/1
  Sum1/1 -> Mux/1, Fcn/1
  Sum2/1 -> Mux/2, Fcn1/1
  Integ2/1 -> Sum2/1, T1/1
  integ1/1 -> T/1, Sum1/1
  T1/1 -> Sum2/2
  T/1 -> Sum1/2
  Product1/1 -> Integ2/1
  Product/1 -> integ1/1
  cos(nwt)/1 -> Product1/2
  sin(nwt)/1 -> Product/1
  Fcn3/1 -> angle/1
  Mux/1 -> Fcn3/1
  Fcn1/1 -> Sum/2
  Fcn/1 -> Sum/1
  Sum/1 -> Fcn2/1
  Constant/1 -> Integ2/2, integ1/2

== system DFIG_FILTER/MODEL (PHASER)/Wind turbine Data acquisition/magnitude positivie seq/Fourier1 ==
  signal : Inport
  Constant : Constant  Value=0
  Fcn : Fcn  Expr=u^2
  Fcn1 : Fcn  Expr=u^2
  Fcn2 : Fcn  Expr=sqrt(u)
  Fcn3 : Fcn  Expr=180/pi*atan2(u[2],u[1])
  Gain1 : Gain  Gain=k*f1  SaturateOnIntegerOverflow=on  OutDataTypeStr=Inherit: Same as input  ParamDataTypeStr=Inherit: Same as input
  Integ2 : Integrator  InitialConditionSource=external
  Mux : Mux  Inputs=2
  Product : Product  InputSameDT=on  SaturateOnIntegerOverflow=on  OutDataTypeStr=Inherit: Same as first input
  Product1 : Product  InputSameDT=on  SaturateOnIntegerOverflow=on  OutDataTypeStr=Inherit: Same as first input
  Sum : Sum  InputSameDT=on  SaturateOnIntegerOverflow=on  OutDataTypeStr=Inherit: Same as first input
  Sum1 : Sum  Inputs=+-  InputSameDT=on  SaturateOnIntegerOverflow=on  OutDataTypeStr=Inherit: Same as first input
  Sum2 : Sum  Inputs=+-  InputSameDT=on  SaturateOnIntegerOverflow=on  OutDataTypeStr=Inherit: Same as first input
  T : TransportDelay  DelayTime=1/f1  BufferSize=2048
  T1 : TransportDelay  DelayTime=1/f1  BufferSize=2048
  cos(nwt) : Sin  Frequency=2*pi*n*f1  Phase=pi/2  SampleTime=0
  integ1 : Integrator  InitialConditionSource=external
  sin(nwt) : Sin  Frequency=2*pi*n*f1  SampleTime=0
  magnitude : Outport  InitialOutput=0  VectorParamsAs1DForOutWhenUnconnected=off
  angle : Outport  Port=2  InitialOutput=0  VectorParamsAs1DForOutWhenUnconnected=off
  wires:
  Fcn2/1 -> magnitude/1
  Gain1/1 -> Product1/1, Product/2
  signal/1 -> Gain1/1
  Sum1/1 -> Mux/1, Fcn/1
  Sum2/1 -> Mux/2, Fcn1/1
  Integ2/1 -> Sum2/1, T1/1
  integ1/1 -> T/1, Sum1/1
  T1/1 -> Sum2/2
  T/1 -> Sum1/2
  Product1/1 -> Integ2/1
  Product/1 -> integ1/1
  cos(nwt)/1 -> Product1/2
  sin(nwt)/1 -> Product/1
  Fcn3/1 -> angle/1
  Mux/1 -> Fcn3/1
  Fcn1/1 -> Sum/2
  Fcn/1 -> Sum/1
  Sum/1 -> Fcn2/1
  Constant/1 -> Integ2/2, integ1/2

== system DFIG_FILTER/MODEL (PHASER)/Wind turbine Data acquisition/magnitude positivie seq/Fourier2 ==
  signal : Inport
  Constant : Constant  Value=0
  Fcn : Fcn  Expr=u^2
  Fcn1 : Fcn  Expr=u^2
  Fcn2 : Fcn  Expr=sqrt(u)
  Fcn3 : Fcn  Expr=180/pi*atan2(u[2],u[1])
  Gain1 : Gain  Gain=k*f1  SaturateOnIntegerOverflow=on  OutDataTypeStr=Inherit: Same as input  ParamDataTypeStr=Inherit: Same as input
  Integ2 : Integrator  InitialConditionSource=external
  Mux : Mux  Inputs=2
  Product : Product  InputSameDT=on  SaturateOnIntegerOverflow=on  OutDataTypeStr=Inherit: Same as first input
  Product1 : Product  InputSameDT=on  SaturateOnIntegerOverflow=on  OutDataTypeStr=Inherit: Same as first input
  Sum : Sum  InputSameDT=on  SaturateOnIntegerOverflow=on  OutDataTypeStr=Inherit: Same as first input
  Sum1 : Sum  Inputs=+-  InputSameDT=on  SaturateOnIntegerOverflow=on  OutDataTypeStr=Inherit: Same as first input
  Sum2 : Sum  Inputs=+-  InputSameDT=on  SaturateOnIntegerOverflow=on  OutDataTypeStr=Inherit: Same as first input
  T : TransportDelay  DelayTime=1/f1  BufferSize=2048
  T1 : TransportDelay  DelayTime=1/f1  BufferSize=2048
  cos(nwt) : Sin  Frequency=2*pi*n*f1  Phase=pi/2  SampleTime=0
  integ1 : Integrator  InitialConditionSource=external
  sin(nwt) : Sin  Frequency=2*pi*n*f1  SampleTime=0
  magnitude : Outport  InitialOutput=0  VectorParamsAs1DForOutWhenUnconnected=off
  angle : Outport  Port=2  InitialOutput=0  VectorParamsAs1DForOutWhenUnconnected=off
  wires:
  Constant/1 -> integ1/2, Integ2/2
  Sum/1 -> Fcn2/1
  Fcn/1 -> Sum/1
  Fcn1/1 -> Sum/2
  Mux/1 -> Fcn3/1
  Fcn3/1 -> angle/1
  sin(nwt)/1 -> Product/1
  cos(nwt)/1 -> Product1/2
  Product/1 -> integ1/1
  Product1/1 -> Integ2/1
  T/1 -> Sum1/2
  T1/1 -> Sum2/2
  integ1/1 -> Sum1/1, T/1
  Integ2/1 -> T1/1, Sum2/1
  Sum2/1 -> Fcn1/1, Mux/2
  Sum1/1 -> Fcn/1, Mux/1
  signal/1 -> Gain1/1
  Gain1/1 -> Product/2, Product1/1
  Fcn2/1 -> magnitude/1

== system DFIG_FILTER/MODEL (PHASER)/Wind turbine Data acquisition1/magnitude positive seq. /Fourier1 ==
  signal : Inport
  Constant : Constant  Value=0
  Fcn : Fcn  Expr=u^2
  Fcn1 : Fcn  Expr=u^2
  Fcn2 : Fcn  Expr=sqrt(u)
  Fcn3 : Fcn  Expr=180/pi*atan2(u[2],u[1])
  Gain1 : Gain  Gain=k*f1  SaturateOnIntegerOverflow=on  OutDataTypeStr=Inherit: Same as input  ParamDataTypeStr=Inherit: Same as input
  Integ2 : Integrator  InitialConditionSource=external
  Mux : Mux  Inputs=2
  Product : Product  InputSameDT=on  SaturateOnIntegerOverflow=on  OutDataTypeStr=Inherit: Same as first input
  Product1 : Product  InputSameDT=on  SaturateOnIntegerOverflow=on  OutDataTypeStr=Inherit: Same as first input
  Sum : Sum  InputSameDT=on  SaturateOnIntegerOverflow=on  OutDataTypeStr=Inherit: Same as first input
  Sum1 : Sum  Inputs=+-  InputSameDT=on  SaturateOnIntegerOverflow=on  OutDataTypeStr=Inherit: Same as first input
  Sum2 : Sum  Inputs=+-  InputSameDT=on  SaturateOnIntegerOverflow=on  OutDataTypeStr=Inherit: Same as first input
  T : TransportDelay  DelayTime=1/f1  BufferSize=2048
  T1 : TransportDelay  DelayTime=1/f1  BufferSize=2048
  cos(nwt) : Sin  Frequency=2*pi*n*f1  Phase=pi/2  SampleTime=0
  integ1 : Integrator  InitialConditionSource=external
  sin(nwt) : Sin  Frequency=2*pi*n*f1  SampleTime=0
  magnitude : Outport  InitialOutput=0  VectorParamsAs1DForOutWhenUnconnected=off
  angle : Outport  Port=2  InitialOutput=0  VectorParamsAs1DForOutWhenUnconnected=off
  wires:
  Constant/1 -> integ1/2, Integ2/2
  Sum/1 -> Fcn2/1
  Fcn/1 -> Sum/1
  Fcn1/1 -> Sum/2
  Mux/1 -> Fcn3/1
  Fcn3/1 -> angle/1
  sin(nwt)/1 -> Product/1
  cos(nwt)/1 -> Product1/2
  Product/1 -> integ1/1
  Product1/1 -> Integ2/1
  T/1 -> Sum1/2
  T1/1 -> Sum2/2
  integ1/1 -> Sum1/1, T/1
  Integ2/1 -> T1/1, Sum2/1
  Sum2/1 -> Fcn1/1, Mux/2
  Sum1/1 -> Fcn/1, Mux/1
  signal/1 -> Gain1/1
  Gain1/1 -> Product/2, Product1/1
  Fcn2/1 -> magnitude/1

== system DFIG_FILTER/MODEL (PHASER)/Wind turbine Data acquisition1/magnitude positive seq. /Fourier2 ==
  signal : Inport
  Constant : Constant  Value=0
  Fcn : Fcn  Expr=u^2
  Fcn1 : Fcn  Expr=u^2
  Fcn2 : Fcn  Expr=sqrt(u)
  Fcn3 : Fcn  Expr=180/pi*atan2(u[2],u[1])
  Gain1 : Gain  Gain=k*f1  SaturateOnIntegerOverflow=on  OutDataTypeStr=Inherit: Same as input  ParamDataTypeStr=Inherit: Same as input
  Integ2 : Integrator  InitialConditionSource=external
  Mux : Mux  Inputs=2
  Product : Product  InputSameDT=on  SaturateOnIntegerOverflow=on  OutDataTypeStr=Inherit: Same as first input
  Product1 : Product  InputSameDT=on  SaturateOnIntegerOverflow=on  OutDataTypeStr=Inherit: Same as first input
  Sum : Sum  InputSameDT=on  SaturateOnIntegerOverflow=on  OutDataTypeStr=Inherit: Same as first input
  Sum1 : Sum  Inputs=+-  InputSameDT=on  SaturateOnIntegerOverflow=on  OutDataTypeStr=Inherit: Same as first input
  Sum2 : Sum  Inputs=+-  InputSameDT=on  SaturateOnIntegerOverflow=on  OutDataTypeStr=Inherit: Same as first input
  T : TransportDelay  DelayTime=1/f1  BufferSize=2048
  T1 : TransportDelay  DelayTime=1/f1  BufferSize=2048
  cos(nwt) : Sin  Frequency=2*pi*n*f1  Phase=pi/2  SampleTime=0
  integ1 : Integrator  InitialConditionSource=external
  sin(nwt) : Sin  Frequency=2*pi*n*f1  SampleTime=0
  magnitude : Outport  InitialOutput=0  VectorParamsAs1DForOutWhenUnconnected=off
  angle : Outport  Port=2  InitialOutput=0  VectorParamsAs1DForOutWhenUnconnected=off
  wires:
  Fcn2/1 -> magnitude/1
  Gain1/1 -> Product1/1, Product/2
  signal/1 -> Gain1/1
  Sum1/1 -> Mux/1, Fcn/1
  Sum2/1 -> Mux/2, Fcn1/1
  Integ2/1 -> Sum2/1, T1/1
  integ1/1 -> T/1, Sum1/1
  T1/1 -> Sum2/2
  T/1 -> Sum1/2
  Product1/1 -> Integ2/1
  Product/1 -> integ1/1
  cos(nwt)/1 -> Product1/2
  sin(nwt)/1 -> Product/1
  Fcn3/1 -> angle/1
  Mux/1 -> Fcn3/1
  Fcn1/1 -> Sum/2
  Fcn/1 -> Sum/1
  Sum/1 -> Fcn2/1
  Constant/1 -> Integ2/2, integ1/2

== system DFIG_FILTER/MODEL (PHASER)/Wind turbine Data acquisition1/magnitude positivie seq/Fourier1 ==
  signal : Inport
  Constant : Constant  Value=0
  Fcn : Fcn  Expr=u^2
  Fcn1 : Fcn  Expr=u^2
  Fcn2 : Fcn  Expr=sqrt(u)
  Fcn3 : Fcn  Expr=180/pi*atan2(u[2],u[1])
  Gain1 : Gain  Gain=k*f1  SaturateOnIntegerOverflow=on  OutDataTypeStr=Inherit: Same as input  ParamDataTypeStr=Inherit: Same as input
  Integ2 : Integrator  InitialConditionSource=external
  Mux : Mux  Inputs=2
  Product : Product  InputSameDT=on  SaturateOnIntegerOverflow=on  OutDataTypeStr=Inherit: Same as first input
  Product1 : Product  InputSameDT=on  SaturateOnIntegerOverflow=on  OutDataTypeStr=Inherit: Same as first input
  Sum : Sum  InputSameDT=on  SaturateOnIntegerOverflow=on  OutDataTypeStr=Inherit: Same as first input
  Sum1 : Sum  Inputs=+-  InputSameDT=on  SaturateOnIntegerOverflow=on  OutDataTypeStr=Inherit: Same as first input
  Sum2 : Sum  Inputs=+-  InputSameDT=on  SaturateOnIntegerOverflow=on  OutDataTypeStr=Inherit: Same as first input
  T : TransportDelay  DelayTime=1/f1  BufferSize=2048
  T1 : TransportDelay  DelayTime=1/f1  BufferSize=2048
  cos(nwt) : Sin  Frequency=2*pi*n*f1  Phase=pi/2  SampleTime=0
  integ1 : Integrator  InitialConditionSource=external
  sin(nwt) : Sin  Frequency=2*pi*n*f1  SampleTime=0
  magnitude : Outport  InitialOutput=0  VectorParamsAs1DForOutWhenUnconnected=off
  angle : Outport  Port=2  InitialOutput=0  VectorParamsAs1DForOutWhenUnconnected=off
  wires:
  Fcn2/1 -> magnitude/1
  Gain1/1 -> Product1/1, Product/2
  signal/1 -> Gain1/1
  Sum1/1 -> Mux/1, Fcn/1
  Sum2/1 -> Mux/2, Fcn1/1
  Integ2/1 -> Sum2/1, T1/1
  integ1/1 -> T/1, Sum1/1
  T1/1 -> Sum2/2
  T/1 -> Sum1/2
  Product1/1 -> Integ2/1
  Product/1 -> integ1/1
  cos(nwt)/1 -> Product1/2
  sin(nwt)/1 -> Product/1
  Fcn3/1 -> angle/1
  Mux/1 -> Fcn3/1
  Fcn1/1 -> Sum/2
  Fcn/1 -> Sum/1
  Sum/1 -> Fcn2/1
  Constant/1 -> Integ2/2, integ1/2

== system DFIG_FILTER/MODEL (PHASER)/Wind turbine Data acquisition1/magnitude positivie seq/Fourier2 ==
  signal : Inport
  Constant : Constant  Value=0
  Fcn : Fcn  Expr=u^2
  Fcn1 : Fcn  Expr=u^2
  Fcn2 : Fcn  Expr=sqrt(u)
  Fcn3 : Fcn  Expr=180/pi*atan2(u[2],u[1])
  Gain1 : Gain  Gain=k*f1  SaturateOnIntegerOverflow=on  OutDataTypeStr=Inherit: Same as input  ParamDataTypeStr=Inherit: Same as input
  Integ2 : Integrator  InitialConditionSource=external
  Mux : Mux  Inputs=2
  Product : Product  InputSameDT=on  SaturateOnIntegerOverflow=on  OutDataTypeStr=Inherit: Same as first input
  Product1 : Product  InputSameDT=on  SaturateOnIntegerOverflow=on  OutDataTypeStr=Inherit: Same as first input
  Sum : Sum  InputSameDT=on  SaturateOnIntegerOverflow=on  OutDataTypeStr=Inherit: Same as first input
  Sum1 : Sum  Inputs=+-  InputSameDT=on  SaturateOnIntegerOverflow=on  OutDataTypeStr=Inherit: Same as first input
  Sum2 : Sum  Inputs=+-  InputSameDT=on  SaturateOnIntegerOverflow=on  OutDataTypeStr=Inherit: Same as first input
  T : TransportDelay  DelayTime=1/f1  BufferSize=2048
  T1 : TransportDelay  DelayTime=1/f1  BufferSize=2048
  cos(nwt) : Sin  Frequency=2*pi*n*f1  Phase=pi/2  SampleTime=0
  integ1 : Integrator  InitialConditionSource=external
  sin(nwt) : Sin  Frequency=2*pi*n*f1  SampleTime=0
  magnitude : Outport  InitialOutput=0  VectorParamsAs1DForOutWhenUnconnected=off
  angle : Outport  Port=2  InitialOutput=0  VectorParamsAs1DForOutWhenUnconnected=off
  wires:
  Constant/1 -> integ1/2, Integ2/2
  Sum/1 -> Fcn2/1
  Fcn/1 -> Sum/1
  Fcn1/1 -> Sum/2
  Mux/1 -> Fcn3/1
  Fcn3/1 -> angle/1
  sin(nwt)/1 -> Product/1
  cos(nwt)/1 -> Product1/2
  Product/1 -> integ1/1
  Product1/1 -> Integ2/1
  T/1 -> Sum1/2
  T1/1 -> Sum2/2
  integ1/1 -> Sum1/1, T/1
  Integ2/1 -> T1/1, Sum2/1
  Sum2/1 -> Fcn1/1, Mux/2
  Sum1/1 -> Fcn/1, Mux/1
  signal/1 -> Gain1/1
  Gain1/1 -> Product/2, Product1/1
  Fcn2/1 -> magnitude/1

== system DFIG_FILTER/MODEL (PHASER)/Wind turbine Data acquisition2/magnitude positive seq. /Fourier1 ==
  signal : Inport
  Constant : Constant  Value=0
  Fcn : Fcn  Expr=u^2
  Fcn1 : Fcn  Expr=u^2
  Fcn2 : Fcn  Expr=sqrt(u)
  Fcn3 : Fcn  Expr=180/pi*atan2(u[2],u[1])
  Gain1 : Gain  Gain=k*f1  SaturateOnIntegerOverflow=on  OutDataTypeStr=Inherit: Same as input  ParamDataTypeStr=Inherit: Same as input
  Integ2 : Integrator  InitialConditionSource=external
  Mux : Mux  Inputs=2
  Product : Product  InputSameDT=on  SaturateOnIntegerOverflow=on  OutDataTypeStr=Inherit: Same as first input
  Product1 : Product  InputSameDT=on  SaturateOnIntegerOverflow=on  OutDataTypeStr=Inherit: Same as first input
  Sum : Sum  InputSameDT=on  SaturateOnIntegerOverflow=on  OutDataTypeStr=Inherit: Same as first input
  Sum1 : Sum  Inputs=+-  InputSameDT=on  SaturateOnIntegerOverflow=on  OutDataTypeStr=Inherit: Same as first input
  Sum2 : Sum  Inputs=+-  InputSameDT=on  SaturateOnIntegerOverflow=on  OutDataTypeStr=Inherit: Same as first input
  T : TransportDelay  DelayTime=1/f1  BufferSize=2048
  T1 : TransportDelay  DelayTime=1/f1  BufferSize=2048
  cos(nwt) : Sin  Frequency=2*pi*n*f1  Phase=pi/2  SampleTime=0
  integ1 : Integrator  InitialConditionSource=external
  sin(nwt) : Sin  Frequency=2*pi*n*f1  SampleTime=0
  magnitude : Outport  InitialOutput=0  VectorParamsAs1DForOutWhenUnconnected=off
  angle : Outport  Port=2  InitialOutput=0  VectorParamsAs1DForOutWhenUnconnected=off
  wires:
  Constant/1 -> integ1/2, Integ2/2
  Sum/1 -> Fcn2/1
  Fcn/1 -> Sum/1
  Fcn1/1 -> Sum/2
  Mux/1 -> Fcn3/1
  Fcn3/1 -> angle/1
  sin(nwt)/1 -> Product/1
  cos(nwt)/1 -> Product1/2
  Product/1 -> integ1/1
  Product1/1 -> Integ2/1
  T/1 -> Sum1/2
  T1/1 -> Sum2/2
  integ1/1 -> Sum1/1, T/1
  Integ2/1 -> T1/1, Sum2/1
  Sum2/1 -> Fcn1/1, Mux/2
  Sum1/1 -> Fcn/1, Mux/1
  signal/1 -> Gain1/1
  Gain1/1 -> Product/2, Product1/1
  Fcn2/1 -> magnitude/1
